simulink model "linearizedTurbine_2023b_mdl"  (R2023b)
settings: Solver=ode4  StartTime=0.0  StopTime=50  FixedStep=.001  RelTol=1e-3
undefined symbols (not defined in the file): F, G, P0
settings Model: Creator=mo780715  LastModifiedBy=mohammadodeh
settings OptimizationCC: ReuseModelBlockBuffer=off

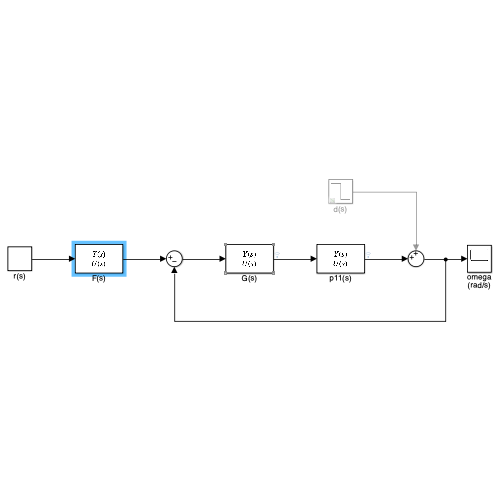
[thumbnail: Simulink's stored preview of the top-level diagram]
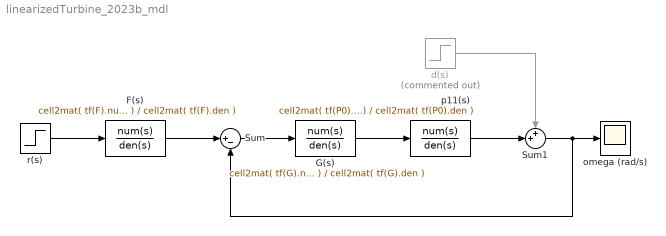
== system linearizedTurbine_2023b_mdl ==
  F(s) : TransferFcn  Numerator=cell2mat( tf(F).num )  Denominator=cell2mat( tf(F).den )
  G(s) : TransferFcn  Numerator=cell2mat( tf(G).num )  Denominator=cell2mat( tf(G).den )  ContinuousStateAttributes='theta'
  Sum : Sum  Inputs=|+-
  Sum1 : Sum  Inputs=++|
  d(s) : Step  Commented=on  Time=35  After=-0.25  SampleTime=0
  omega (rad/s) : Scope
  p11(s) : TransferFcn  Numerator=cell2mat( tf(P0).num )  Denominator=cell2mat( tf(P0).den )  ContinuousStateAttributes='theta'
  r(s) : Step  Time=5  After=0.5  SampleTime=0
  wires:
  Sum1/1 -> omega (rad/s)/1, Sum/2
  F(s)/1 -> Sum/1
  Sum/1 -> G(s)/1
  r(s)/1 -> F(s)/1
  p11(s)/1 -> Sum1/2
  d(s)/1 -> Sum1/1
  G(s)/1 -> p11(s)/1
